simulink model "modified_controller"  (R2018a)
settings: Solver=VariableStepAuto  StartTime=0.0  StopTime=ttotal  RelTol=1e-3
values from neighbouring files (symbols this model uses):
  b = 0    [e_11.m]    (also in e_12.m = 0.025; e_13.m; lab2.m)
  f = 0    [e_11.m]    (also in e_12.m = 1; e_13.m = 1; lab2.m = 1)
  k1 = 1/yl    [cont_10.m]    (also in e_10.m = 1/yl(n); e_11.m = 5; e_12.m = 5; e_13.m = 5)
  k2 = sqrt(2*k1)    [cont_10.m]    (also in e_10.m; e_11.m; e_12.m; e_13.m)
  Ref = 0    [e_11.m]    (also in e_12.m; lab2.m)
  yl = [0, 0.2, 0.4]    [e_10.m]    (also in e_11.m = 0.2; e_12.m = 0.2; e_13.m = 0.2; lab2.m = 0.2)
undefined symbols (not defined in the file or in its folder): sgn
settings Model: Creator=Carlos  LastModifiedBy=Carlos

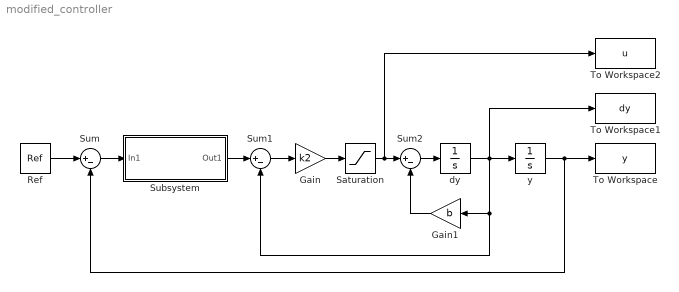
== system modified_controller ==
  Gain : Gain  Gain=k2
  Gain1 : Gain  Gain=b
  Ref : Constant  Value=Ref
  Saturation : Saturate  UpperLimit=1  LowerLimit=-1  LinearizeAsGain=off  ZeroCross=off
  Subsystem : Subsystem
  Sum : Sum  Inputs=|+-
  Sum1 : Sum  Inputs=|+-
  Sum2 : Sum  Inputs=|+-
  To Workspace : ToWorkspace  VariableName=y  SampleTime=-1
  To Workspace1 : ToWorkspace  VariableName=dy  SampleTime=-1
  To Workspace2 : ToWorkspace  VariableName=u  SampleTime=-1
  dy : Integrator
  y : Integrator  InitialCondition=1
  wires:
  Ref/1 -> Sum/1
  Sum/1 -> Subsystem/1(In1)
  Subsystem/1(Out1) -> Sum1/1
  Sum1/1 -> Gain/1
  Gain/1 -> Saturation/1
  dy/1 -> To Workspace1/1, Gain1/1, Sum1/2, y/1
  y/1 -> Sum/2, To Workspace/1
  Saturation/1 -> To Workspace2/1, Sum2/1
  Sum2/1 -> dy/1
  Gain1/1 -> Sum2/2

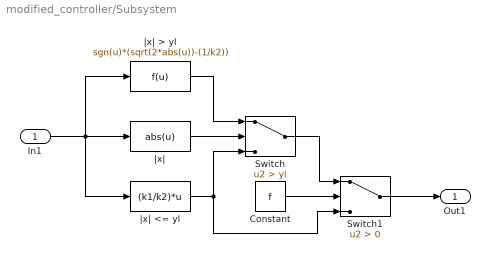
== system modified_controller/Subsystem ==
  In1 : Inport
  Constant : Constant  Value=f
  Switch : Switch  Criteria=u2 > Threshold  Threshold=yl  ZeroCross=off
  Switch1 : Switch  Criteria=u2 > Threshold  ZeroCross=off
  |x| : Fcn  Expr=abs(u)
  |x| <= yl : Fcn  Expr=(k1/k2)*u
  |x| > yl : Fcn  Expr=sgn(u)*(sqrt(2*abs(u))-(1/k2))
  Out1 : Outport
  wires:
  In1/1 -> |x| <= yl/1, |x| > yl/1, |x|/1
  |x|/1 -> Switch/2
  |x| > yl/1 -> Switch/1
  |x| <= yl/1 -> Switch1/3, Switch/3
  Switch1/1 -> Out1/1
  Constant/1 -> Switch1/2
  Switch/1 -> Switch1/1
